simulink model "isolatedInjectorTest"  (R2020b)
settings: Solver=VariableStepAuto  StartTime=0.0  StopTime=10.0  RelTol=1e-3
libraries: fl_lib x5, nesl_utility x2
settings Model: Creator=Edward  LastModifiedBy=Edward

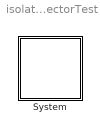
== system isolatedInjectorTest ==
  System : Subsystem  mask{upstreamPressure=40e5}
      mask prompts: upstreamPressure "Upstream Pressure (Pa)"

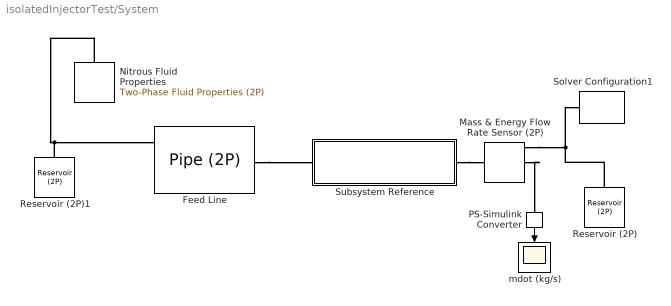
== system isolatedInjectorTest/System ==
  Feed Line : fl_lib/Two-Phase Fluid/Elements/Pipe (2P)  length=10 cm  area=1.96e-5 m^2  Dh=5e-3 m  length_add=10 cm  roughness=15e-6 m  Re_lam=2000  Re_tur=4000  shape_factor=64  Nu_lam=3.66  inertia=simscape.enum.onoff.on  energy_spec=foundation.enum.energy_spec.temperature  p_init=upstreamPressure Pa  T_init=293.15 K  x_init=0.5  alpha_init=0.5  h_init=1500 kJ/kg  u_init=1500 kJ/kg  mdot_init=0 kg/s  time_constant=0.1 s
      settings: SourceProductBaseCode=SS  InternalSimscapePortConfiguration="{\"Bottom\":[],\"Left\":[{\"id\":\"A\",\"label\":\"A\",\"type\":\"foundation.two_phase_fluid.two_phase_fluid\"},{\"id\":\"H\",\"label\":\"H\",\"type\":\"foundation.thermal.thermal\"}],\"Right\":[{\"id\":\"B\",\"label\":\"B\",\"type\":\"foundation.two_phase_fluid.two_phase_fluid\"}],\"Top\":[]}"
  Mass & Energy Flow Rate Sensor (2P) : fl_lib/Two-Phase Fluid/Sensors/Mass & Energy Flow Rate Sensor (2P)
      settings: SourceProductBaseCode=SS  InternalSimscapePortConfiguration="{\"Bottom\":[],\"Left\":[{\"id\":\"A\",\"label\":\"A\",\"type\":\"foundation.two_phase_fluid.two_phase_fluid\"}],\"Right\":[{\"id\":\"B\",\"label\":\"B\",\"type\":\"foundation.two_phase_fluid.two_phase_fluid\"},{\"id\":\"M\",\"label\":\"M\",\"type\":\"output\"},{\"id\":\"PHI\",\"label\":\"Phi\",\"type\":\"output\"}],\"Top\":[]}"
  Nitrous Fluid Properties : fl_lib/Two-Phase Fluid/Utilities/Two-Phase Fluid Properties (2P)  u_min=sim.nitrousFluidTable.u_min kJ/kg  u_max=sim.nitrousFluidTable.u_max kJ/kg  unorm_liq=sim.nitrousFluidTable.liquid.unorm  unorm_vap=sim.nitrousFluidTable.vapor.unorm  p_TLU=sim.nitrousFluidTable.p MPa  v_liq=sim.nitrousFluidTable.liquid.v m^3/kg  v_vap=sim.nitrousFluidTable.vapor.v m^3/kg  s_liq=sim.nitrousFluidTable.liquid.s kJ/kg/K  s_vap=sim.nitrousFluidTable.vapor.s kJ/kg/K  T_liq=sim.nitrousFluidTable.liquid.T K  T_vap=sim.nitrousFluidTable.vapor.T K  nu_liq=sim.nitrousFluidTable.liquid.nu mm^2/s  nu_vap=sim.nitrousFluidTable.vapor.nu mm^2/s  k_liq=sim.nitrousFluidTable.liquid.k W/(m*K)  k_vap=sim.nitrousFluidTable.vapor.k W/(m*K)  Pr_liq=sim.nitrousFluidTable.liquid.Pr  Pr_vap=sim.nitrousFluidTable.vapor.Pr  u_sat_liq=sim.nitrousFluidTable.liquid.u_sat kJ/kg  u_sat_vap=sim.nitrousFluidTable.vapor.u_sat kJ/kg  p_crit=sim.nitrousFluidTable.p_crit MPa  critical_region=foundation.enum.critical_region.clip  p_crit_fraction=0.12  p_atm=0.101325 MPa  q_rev=0.01 Pa
      settings: SourceProductBaseCode=SS  InternalSimscapePortConfiguration="{\"Bottom\":[],\"Left\":[],\"Right\":[{\"id\":\"A\",\"label\":\"\",\"type\":\"foundation.two_phase_fluid.two_phase_fluid\"}],\"Top\":[]}"
  PS-Simulink Converter : nesl_utility/PS-Simulink Converter  PhysicalDomain=network_engine_domain  SubClassName=ps_output  LeftPortType=input  RightPortType=output  PseudoPeriodic=off  Frequencies=[]  Unit=inherit  AffineConversion=off
  Reservoir (2P) : fl_lib/Two-Phase Fluid/Elements/Reservoir (2P)  pressure_spec=foundation.enum.pressure_spec.specified  reservoir_pressure=30e5 Pa  energy_spec=foundation.enum.energy_spec.temperature  reservoir_temperature=293.15 K  reservoir_quality=0.5  reservoir_void_fraction=0.5  reservoir_enthalpy=1500 kJ/kg  reservoir_internal_energy=1500 kJ/kg  area_A=0.01 m^2
      settings: SourceProductBaseCode=SS
  Reservoir (2P)1 : fl_lib/Two-Phase Fluid/Elements/Reservoir (2P)  pressure_spec=foundation.enum.pressure_spec.specified  reservoir_pressure=upstreamPressure Pa  energy_spec=foundation.enum.energy_spec.quality  reservoir_temperature=293.15 K  reservoir_quality=0  reservoir_void_fraction=0.5  reservoir_enthalpy=1500 kJ/kg  reservoir_internal_energy=1500 kJ/kg  area_A=0.01 m^2
      settings: SourceProductBaseCode=SS
  Solver Configuration1 : nesl_utility/Solver Configuration  PhysicalDomain=network_engine_domain  SubClassName=solver  LeftPortType=input  RightPortType=generic  Tones=[]  Harmonics=[]  SimulateNoise=off  Profile=off  UseLocalSampling=off  EnableSwitchedLinearOptims=on  FrequencyDomain=off  UseCCode=off  RelTol=0.001  AbsTol=1e-06  MinStep=1e-09  ToWorkspace=off  RevertToSquareIcSolve=off  NumHomotopyIterations=100  PhasorMode=off  PhasorModeNumHarmonics=1  DoDC=off  ResidualTolerance=1e-9  UseLocalSolver=off  LocalSolverChoice=NE_BACKWARD_EULER_ADVANCER  LocalSolverSampleTime=0.001  DoFixedCost=off  MaxNonlinIter=3  MaxModeIter=2  ComputeImpulses=off  ImpulseIterations=2  LinearAlgebra=auto  EquationFormulation=NE_TIME_EF  DelaysMemoryBudget=1024  AutomaticFiltering=on  FilteringTimeConstant=0.001  PartitionStorageMethod=AS_NEEDED  PartitionMemoryBudget=1024  PartitionMethod=ROBUST
  Subsystem Reference : Subsystem  ReferencedSubsystem=Injector  dischargeCoeff=0.64
  mdot (kg/s) : Scope
  wires:
  PS-Simulink Converter/1 -> mdot (kg/s)/1
  connections:
  Reservoir (2P)/LConn1 -- Mass & Energy Flow Rate Sensor (2P)/RConn1 -- Solver Configuration1/RConn1
  Feed Line/RConn1 -- Subsystem Reference/LConn1
  Reservoir (2P)1/LConn1 -- Feed Line/LConn1 -- Nitrous Fluid Properties/RConn1
  Subsystem Reference/RConn1 -- Mass & Energy Flow Rate Sensor (2P)/LConn1
  Mass & Energy Flow Rate Sensor (2P)/RConn2 -- PS-Simulink Converter/LConn1
